simulink model "fine_delay_core"  (R2012b)
settings: Solver=ode45  StartTime=0.0  StopTime=10.0  RelTol=1e-3
libraries: xbsIndex_r4 x410, casper_library_misc x16, casper_library_multipliers x8
(part 2 of 4)

== system fine_delay_core/fd_fs0/fd_fs0/rotate0 ==
  sync : Inport
  x : Inport  Port=2
  a0 : Inport  Port=3
  a1 : Inport  Port=4
  din : Inport  Port=5
  Convert : xbsIndex_r4/Convert  gui_display_data_type=Fixed-point  arith_type="Signed  (2's comp)"  n_bits=data_bit_width  bin_pt=data_bit_width-1  float_type=Single  exp_bits=8  fraction_bits=24  quantization="Round  (unbiased: Even Values)"  overflow=Wrap  en=off  latency=conv_latency  dbl_ovrd=off  pipeline=on  block_type=convert
      settings: block_version=10.1.3
  Convert1 : xbsIndex_r4/Convert  gui_display_data_type=Fixed-point  arith_type="Signed  (2's comp)"  n_bits=data_bit_width  bin_pt=data_bit_width-1  float_type=Single  exp_bits=8  fraction_bits=24  quantization="Round  (unbiased: Even Values)"  overflow=Wrap  en=off  latency=conv_latency  dbl_ovrd=off  pipeline=on  block_type=convert
      settings: block_version=10.1.3
  Convert8 : xbsIndex_r4/Convert  gui_display_data_type=Fixed-point  arith_type="Signed  (2's comp)"  n_bits=lookup_bit_width  bin_pt=lookup_bit_width-1  float_type=Single  exp_bits=8  fraction_bits=24  quantization="Round  (unbiased: +/- Inf)"  overflow=Wrap  en=off  latency=conv_latency  dbl_ovrd=off  pipeline=on  block_type=convert
      settings: block_version=10.1.3
  Delay10 : xbsIndex_r4/Delay  rst=off  infoeditControl=Selection of Reset will increase slice count due to use of real FFs and instead of SRLs  en=off  latency=bram_latency  dbl_ovrd=off  reg_retiming=on  block_type=delay
  Delay13 : xbsIndex_r4/Delay  rst=off  infoeditControl=Selection of Reset will increase slice count due to use of real FFs and instead of SRLs  en=off  latency=conv_latency  dbl_ovrd=off  reg_retiming=on  block_type=delay
  Delay3 : xbsIndex_r4/Delay  rst=off  infoeditControl=Selection of Reset will increase slice count due to use of real FFs and instead of SRLs  en=off  latency=bram_latency  dbl_ovrd=off  reg_retiming=on  block_type=delay
  Delay6 : xbsIndex_r4/Delay  rst=off  infoeditControl=Selection of Reset will increase slice count due to use of real FFs and instead of SRLs  en=off  latency=mult_latency+add_latency+conv_latency  dbl_ovrd=off  reg_retiming=on  block_type=delay
  Delay9 : xbsIndex_r4/Delay  rst=off  infoeditControl=Selection of Reset will increase slice count due to use of real FFs and instead of SRLs  en=off  latency=add_latency+mult_latency+conv_latency  dbl_ovrd=off  reg_retiming=on  block_type=delay
  Reinterpret11 : xbsIndex_r4/Reinterpret  force_arith_type=on  arith_type=Unsigned  force_bin_pt=on  bin_pt=0  block_type=reinterpret
      settings: infoedit="Changes signal type without altering the binary representation.   You can changed the signal between signed and unsigned, and relocate the binary point.<br><br>Hardware notes: In hardware this block costs nothing.<br><br>Example:  Suppose the input is 6 bits wide, signed, with 2 fractional bits, and the output is forced to unsigned with 0 fractional bits.  Then an input of -2.0 (1110.00 in binary 2's complement) becomes an output of 56 (111000 in binary)."  block_version=10.1.3
  c_to_ri : casper_library_misc/c_to_ri  n_bits=data_bit_width  bin_pt=data_bit_width-1
  cmult_dsp48e : casper_library_multipliers/cmult_dsp48e  n_bits_a=18  bin_pt_a=17  n_bits_b=18  bin_pt_b=17  conjugated=off  full_precision=on  n_bits_c=37  bin_pt_c=34  quantization=Truncate  overflow=Wrap  cast_latency=0
      settings: AttributesFormatString=|
      | 18_17 * 18_17 ==> 37_34
      | Latency=4
  polynomial0 : Subsystem  mask(polynomial){order=1, mult_latency=mult_latency, add_latency=add_latency, bit_width_out=lookup_bit_width+fft_len, bin_pt_out=fft_len}
      mask prompts: order "Order of polynomial"; mult_latency "Multiplier latency"; add_latency "Add latency"; bit_width_out "Output bit width"; bin_pt_out "Output binary point"
      settings: AttributesFormatString=latency 6
  ri_to_c : casper_library_misc/ri_to_c
  sincos0 : Subsystem  AncestorBlock=casper_library_downconverter/sincos  mask(sincos){func=sine and cosine, neg_sin=off, neg_cos=off, symmetric=off, handle_sync=on, depth_bits=lookup_bit_width, bit_width=mix_bits, bram_latency=bram_latency}
      mask prompts: func "Function"; neg_sin "Negative sine"; neg_cos "Negative cosine"; symmetric "Symmetric output"; handle_sync "Handle sync"; depth_bits "Lookup table depth (2^?)"; bit_width "Output bit width"; bram_latency "BRAM latency"
      mask init:
      | sincos_init(gcb, ...
      |     'func', func, ...
      |     'neg_sin', neg_sin, ...
      |     'neg_cos', neg_cos, ...
      |     'symmetric', symmetric, ...
      |     'handle_sync', handle_sync, ...
      |     'depth_bits', depth_bits, ...
      |     'bit_width', bit_width, ...
      |     'bram_latency', bram_latency);
      mask TypeOptions func: cosine | sine | sine and cosine
  sync_out : Outport
  dout : Outport  Port=2
  wires:
  polynomial0/2(a0x^0+a1x^1) -> Convert8/1
  polynomial0/1(sync_out) -> Delay13/1
  Reinterpret11/1 -> sincos0/2(theta)
  sincos0/1(sync_out) -> Delay6/1
  cmult_dsp48e/1 -> Convert/1
  cmult_dsp48e/2 -> Convert1/1
  Convert/1 -> ri_to_c/1
  Convert1/1 -> ri_to_c/2
  sincos0/3(cos) -> cmult_dsp48e/1
  sincos0/2(sine) -> cmult_dsp48e/2
  c_to_ri/1 -> Delay10/1
  Delay10/1 -> cmult_dsp48e/3
  c_to_ri/2 -> Delay3/1
  Delay3/1 -> cmult_dsp48e/4
  Delay9/1 -> c_to_ri/1
  Delay13/1 -> sincos0/1(sync_in)
  Convert8/1 -> Reinterpret11/1
  sync/1 -> polynomial0/1(sync_in)
  Delay6/1 -> sync_out/1
  x/1 -> polynomial0/2(x)
  a0/1 -> polynomial0/3(a0)
  a1/1 -> polynomial0/4(a1)
  ri_to_c/1 -> dout/1
  din/1 -> Delay9/1

== system fine_delay_core/fd_fs0/fd_fs0/rotate1 ==
  sync : Inport
  x : Inport  Port=2
  a0 : Inport  Port=3
  a1 : Inport  Port=4
  din : Inport  Port=5
  Convert : xbsIndex_r4/Convert  gui_display_data_type=Fixed-point  arith_type="Signed  (2's comp)"  n_bits=data_bit_width  bin_pt=data_bit_width-1  float_type=Single  exp_bits=8  fraction_bits=24  quantization="Round  (unbiased: Even Values)"  overflow=Wrap  en=off  latency=conv_latency  dbl_ovrd=off  pipeline=on  block_type=convert
      settings: block_version=10.1.3
  Convert1 : xbsIndex_r4/Convert  gui_display_data_type=Fixed-point  arith_type="Signed  (2's comp)"  n_bits=data_bit_width  bin_pt=data_bit_width-1  float_type=Single  exp_bits=8  fraction_bits=24  quantization="Round  (unbiased: Even Values)"  overflow=Wrap  en=off  latency=conv_latency  dbl_ovrd=off  pipeline=on  block_type=convert
      settings: block_version=10.1.3
  Convert8 : xbsIndex_r4/Convert  gui_display_data_type=Fixed-point  arith_type="Signed  (2's comp)"  n_bits=lookup_bit_width  bin_pt=lookup_bit_width-1  float_type=Single  exp_bits=8  fraction_bits=24  quantization="Round  (unbiased: +/- Inf)"  overflow=Wrap  en=off  latency=conv_latency  dbl_ovrd=off  pipeline=on  block_type=convert
      settings: block_version=10.1.3
  Delay10 : xbsIndex_r4/Delay  rst=off  infoeditControl=Selection of Reset will increase slice count due to use of real FFs and instead of SRLs  en=off  latency=bram_latency  dbl_ovrd=off  reg_retiming=on  block_type=delay
  Delay13 : xbsIndex_r4/Delay  rst=off  infoeditControl=Selection of Reset will increase slice count due to use of real FFs and instead of SRLs  en=off  latency=conv_latency  dbl_ovrd=off  reg_retiming=on  block_type=delay
  Delay3 : xbsIndex_r4/Delay  rst=off  infoeditControl=Selection of Reset will increase slice count due to use of real FFs and instead of SRLs  en=off  latency=bram_latency  dbl_ovrd=off  reg_retiming=on  block_type=delay
  Delay6 : xbsIndex_r4/Delay  rst=off  infoeditControl=Selection of Reset will increase slice count due to use of real FFs and instead of SRLs  en=off  latency=mult_latency+add_latency+conv_latency  dbl_ovrd=off  reg_retiming=on  block_type=delay
  Delay9 : xbsIndex_r4/Delay  rst=off  infoeditControl=Selection of Reset will increase slice count due to use of real FFs and instead of SRLs  en=off  latency=add_latency+mult_latency+conv_latency  dbl_ovrd=off  reg_retiming=on  block_type=delay
  Reinterpret11 : xbsIndex_r4/Reinterpret  force_arith_type=on  arith_type=Unsigned  force_bin_pt=on  bin_pt=0  block_type=reinterpret
      settings: infoedit="Changes signal type without altering the binary representation.   You can changed the signal between signed and unsigned, and relocate the binary point.<br><br>Hardware notes: In hardware this block costs nothing.<br><br>Example:  Suppose the input is 6 bits wide, signed, with 2 fractional bits, and the output is forced to unsigned with 0 fractional bits.  Then an input of -2.0 (1110.00 in binary 2's complement) becomes an output of 56 (111000 in binary)."  block_version=10.1.3
  c_to_ri : casper_library_misc/c_to_ri  n_bits=data_bit_width  bin_pt=data_bit_width-1
  cmult_dsp48e : casper_library_multipliers/cmult_dsp48e  n_bits_a=18  bin_pt_a=17  n_bits_b=18  bin_pt_b=17  conjugated=off  full_precision=on  n_bits_c=37  bin_pt_c=34  quantization=Truncate  overflow=Wrap  cast_latency=0
      settings: AttributesFormatString=|
      | 18_17 * 18_17 ==> 37_34
      | Latency=4
  polynomial0 : Subsystem  mask(polynomial){order=1, mult_latency=mult_latency, add_latency=add_latency, bit_width_out=lookup_bit_width+fft_len, bin_pt_out=fft_len}
      mask prompts: order "Order of polynomial"; mult_latency "Multiplier latency"; add_latency "Add latency"; bit_width_out "Output bit width"; bin_pt_out "Output binary point"
      settings: AttributesFormatString=latency 6
  ri_to_c : casper_library_misc/ri_to_c
  sincos0 : Subsystem  AncestorBlock=casper_library_downconverter/sincos  mask(sincos){func=sine and cosine, neg_sin=off, neg_cos=off, symmetric=off, handle_sync=on, depth_bits=lookup_bit_width, bit_width=mix_bits, bram_latency=bram_latency}
      mask prompts: func "Function"; neg_sin "Negative sine"; neg_cos "Negative cosine"; symmetric "Symmetric output"; handle_sync "Handle sync"; depth_bits "Lookup table depth (2^?)"; bit_width "Output bit width"; bram_latency "BRAM latency"
      mask init: same as fine_delay_core/fd_fs0/fd_fs0/rotate0/sincos0
      mask TypeOptions func: cosine | sine | sine and cosine
  sync_out : Outport
  dout : Outport  Port=2
  wires:
  din/1 -> Delay9/1
  ri_to_c/1 -> dout/1
  a1/1 -> polynomial0/4(a1)
  a0/1 -> polynomial0/3(a0)
  x/1 -> polynomial0/2(x)
  Delay6/1 -> sync_out/1
  sync/1 -> polynomial0/1(sync_in)
  Convert8/1 -> Reinterpret11/1
  Delay13/1 -> sincos0/1(sync_in)
  Delay9/1 -> c_to_ri/1
  Delay3/1 -> cmult_dsp48e/4
  c_to_ri/2 -> Delay3/1
  Delay10/1 -> cmult_dsp48e/3
  c_to_ri/1 -> Delay10/1
  sincos0/2(sine) -> cmult_dsp48e/2
  sincos0/3(cos) -> cmult_dsp48e/1
  Convert1/1 -> ri_to_c/2
  Convert/1 -> ri_to_c/1
  cmult_dsp48e/2 -> Convert1/1
  cmult_dsp48e/1 -> Convert/1
  sincos0/1(sync_out) -> Delay6/1
  Reinterpret11/1 -> sincos0/2(theta)
  polynomial0/1(sync_out) -> Delay13/1
  polynomial0/2(a0x^0+a1x^1) -> Convert8/1

== system fine_delay_core/fd_fs0/fd_fs0/rotate2 ==
  sync : Inport
  x : Inport  Port=2
  a0 : Inport  Port=3
  a1 : Inport  Port=4
  din : Inport  Port=5
  Convert : xbsIndex_r4/Convert  gui_display_data_type=Fixed-point  arith_type="Signed  (2's comp)"  n_bits=data_bit_width  bin_pt=data_bit_width-1  float_type=Single  exp_bits=8  fraction_bits=24  quantization="Round  (unbiased: Even Values)"  overflow=Wrap  en=off  latency=conv_latency  dbl_ovrd=off  pipeline=on  block_type=convert
      settings: block_version=10.1.3
  Convert1 : xbsIndex_r4/Convert  gui_display_data_type=Fixed-point  arith_type="Signed  (2's comp)"  n_bits=data_bit_width  bin_pt=data_bit_width-1  float_type=Single  exp_bits=8  fraction_bits=24  quantization="Round  (unbiased: Even Values)"  overflow=Wrap  en=off  latency=conv_latency  dbl_ovrd=off  pipeline=on  block_type=convert
      settings: block_version=10.1.3
  Convert8 : xbsIndex_r4/Convert  gui_display_data_type=Fixed-point  arith_type="Signed  (2's comp)"  n_bits=lookup_bit_width  bin_pt=lookup_bit_width-1  float_type=Single  exp_bits=8  fraction_bits=24  quantization="Round  (unbiased: +/- Inf)"  overflow=Wrap  en=off  latency=conv_latency  dbl_ovrd=off  pipeline=on  block_type=convert
      settings: block_version=10.1.3
  Delay10 : xbsIndex_r4/Delay  rst=off  infoeditControl=Selection of Reset will increase slice count due to use of real FFs and instead of SRLs  en=off  latency=bram_latency  dbl_ovrd=off  reg_retiming=on  block_type=delay
  Delay13 : xbsIndex_r4/Delay  rst=off  infoeditControl=Selection of Reset will increase slice count due to use of real FFs and instead of SRLs  en=off  latency=conv_latency  dbl_ovrd=off  reg_retiming=on  block_type=delay
  Delay3 : xbsIndex_r4/Delay  rst=off  infoeditControl=Selection of Reset will increase slice count due to use of real FFs and instead of SRLs  en=off  latency=bram_latency  dbl_ovrd=off  reg_retiming=on  block_type=delay
  Delay6 : xbsIndex_r4/Delay  rst=off  infoeditControl=Selection of Reset will increase slice count due to use of real FFs and instead of SRLs  en=off  latency=mult_latency+add_latency+conv_latency  dbl_ovrd=off  reg_retiming=on  block_type=delay
  Delay9 : xbsIndex_r4/Delay  rst=off  infoeditControl=Selection of Reset will increase slice count due to use of real FFs and instead of SRLs  en=off  latency=add_latency+mult_latency+conv_latency  dbl_ovrd=off  reg_retiming=on  block_type=delay
  Reinterpret11 : xbsIndex_r4/Reinterpret  force_arith_type=on  arith_type=Unsigned  force_bin_pt=on  bin_pt=0  block_type=reinterpret
      settings: infoedit="Changes signal type without altering the binary representation.   You can changed the signal between signed and unsigned, and relocate the binary point.<br><br>Hardware notes: In hardware this block costs nothing.<br><br>Example:  Suppose the input is 6 bits wide, signed, with 2 fractional bits, and the output is forced to unsigned with 0 fractional bits.  Then an input of -2.0 (1110.00 in binary 2's complement) becomes an output of 56 (111000 in binary)."  block_version=10.1.3
  c_to_ri : casper_library_misc/c_to_ri  n_bits=data_bit_width  bin_pt=data_bit_width-1
  cmult_dsp48e : casper_library_multipliers/cmult_dsp48e  n_bits_a=18  bin_pt_a=17  n_bits_b=18  bin_pt_b=17  conjugated=off  full_precision=on  n_bits_c=37  bin_pt_c=34  quantization=Truncate  overflow=Wrap  cast_latency=0
      settings: AttributesFormatString=|
      | 18_17 * 18_17 ==> 37_34
      | Latency=4
  polynomial0 : Subsystem  mask(polynomial){order=1, mult_latency=mult_latency, add_latency=add_latency, bit_width_out=lookup_bit_width+fft_len, bin_pt_out=fft_len}
      mask prompts: order "Order of polynomial"; mult_latency "Multiplier latency"; add_latency "Add latency"; bit_width_out "Output bit width"; bin_pt_out "Output binary point"
      settings: AttributesFormatString=latency 6
  ri_to_c : casper_library_misc/ri_to_c
  sincos0 : Subsystem  AncestorBlock=casper_library_downconverter/sincos  mask(sincos){func=sine and cosine, neg_sin=off, neg_cos=off, symmetric=off, handle_sync=on, depth_bits=lookup_bit_width, bit_width=mix_bits, bram_latency=bram_latency}
      mask prompts: func "Function"; neg_sin "Negative sine"; neg_cos "Negative cosine"; symmetric "Symmetric output"; handle_sync "Handle sync"; depth_bits "Lookup table depth (2^?)"; bit_width "Output bit width"; bram_latency "BRAM latency"
      mask init: same as fine_delay_core/fd_fs0/fd_fs0/rotate0/sincos0
      mask TypeOptions func: cosine | sine | sine and cosine
  sync_out : Outport
  dout : Outport  Port=2
  wires:
  din/1 -> Delay9/1
  ri_to_c/1 -> dout/1
  a1/1 -> polynomial0/4(a1)
  a0/1 -> polynomial0/3(a0)
  x/1 -> polynomial0/2(x)
  Delay6/1 -> sync_out/1
  sync/1 -> polynomial0/1(sync_in)
  Convert8/1 -> Reinterpret11/1
  Delay13/1 -> sincos0/1(sync_in)
  Delay9/1 -> c_to_ri/1
  Delay3/1 -> cmult_dsp48e/4
  c_to_ri/2 -> Delay3/1
  Delay10/1 -> cmult_dsp48e/3
  c_to_ri/1 -> Delay10/1
  sincos0/2(sine) -> cmult_dsp48e/2
  sincos0/3(cos) -> cmult_dsp48e/1
  Convert1/1 -> ri_to_c/2
  Convert/1 -> ri_to_c/1
  cmult_dsp48e/2 -> Convert1/1
  cmult_dsp48e/1 -> Convert/1
  sincos0/1(sync_out) -> Delay6/1
  Reinterpret11/1 -> sincos0/2(theta)
  polynomial0/1(sync_out) -> Delay13/1
  polynomial0/2(a0x^0+a1x^1) -> Convert8/1

== system fine_delay_core/fd_fs0/fd_fs0/rotate3 ==
  sync : Inport
  x : Inport  Port=2
  a0 : Inport  Port=3
  a1 : Inport  Port=4
  din : Inport  Port=5
  Convert : xbsIndex_r4/Convert  gui_display_data_type=Fixed-point  arith_type="Signed  (2's comp)"  n_bits=data_bit_width  bin_pt=data_bit_width-1  float_type=Single  exp_bits=8  fraction_bits=24  quantization="Round  (unbiased: Even Values)"  overflow=Wrap  en=off  latency=conv_latency  dbl_ovrd=off  pipeline=on  block_type=convert
      settings: block_version=10.1.3
  Convert1 : xbsIndex_r4/Convert  gui_display_data_type=Fixed-point  arith_type="Signed  (2's comp)"  n_bits=data_bit_width  bin_pt=data_bit_width-1  float_type=Single  exp_bits=8  fraction_bits=24  quantization="Round  (unbiased: Even Values)"  overflow=Wrap  en=off  latency=conv_latency  dbl_ovrd=off  pipeline=on  block_type=convert
      settings: block_version=10.1.3
  Convert8 : xbsIndex_r4/Convert  gui_display_data_type=Fixed-point  arith_type="Signed  (2's comp)"  n_bits=lookup_bit_width  bin_pt=lookup_bit_width-1  float_type=Single  exp_bits=8  fraction_bits=24  quantization="Round  (unbiased: +/- Inf)"  overflow=Wrap  en=off  latency=conv_latency  dbl_ovrd=off  pipeline=on  block_type=convert
      settings: block_version=10.1.3
  Delay10 : xbsIndex_r4/Delay  rst=off  infoeditControl=Selection of Reset will increase slice count due to use of real FFs and instead of SRLs  en=off  latency=bram_latency  dbl_ovrd=off  reg_retiming=on  block_type=delay
  Delay13 : xbsIndex_r4/Delay  rst=off  infoeditControl=Selection of Reset will increase slice count due to use of real FFs and instead of SRLs  en=off  latency=conv_latency  dbl_ovrd=off  reg_retiming=on  block_type=delay
  Delay3 : xbsIndex_r4/Delay  rst=off  infoeditControl=Selection of Reset will increase slice count due to use of real FFs and instead of SRLs  en=off  latency=bram_latency  dbl_ovrd=off  reg_retiming=on  block_type=delay
  Delay6 : xbsIndex_r4/Delay  rst=off  infoeditControl=Selection of Reset will increase slice count due to use of real FFs and instead of SRLs  en=off  latency=mult_latency+add_latency+conv_latency  dbl_ovrd=off  reg_retiming=on  block_type=delay
  Delay9 : xbsIndex_r4/Delay  rst=off  infoeditControl=Selection of Reset will increase slice count due to use of real FFs and instead of SRLs  en=off  latency=add_latency+mult_latency+conv_latency  dbl_ovrd=off  reg_retiming=on  block_type=delay
  Reinterpret11 : xbsIndex_r4/Reinterpret  force_arith_type=on  arith_type=Unsigned  force_bin_pt=on  bin_pt=0  block_type=reinterpret
      settings: infoedit="Changes signal type without altering the binary representation.   You can changed the signal between signed and unsigned, and relocate the binary point.<br><br>Hardware notes: In hardware this block costs nothing.<br><br>Example:  Suppose the input is 6 bits wide, signed, with 2 fractional bits, and the output is forced to unsigned with 0 fractional bits.  Then an input of -2.0 (1110.00 in binary 2's complement) becomes an output of 56 (111000 in binary)."  block_version=10.1.3
  c_to_ri : casper_library_misc/c_to_ri  n_bits=data_bit_width  bin_pt=data_bit_width-1
  cmult_dsp48e : casper_library_multipliers/cmult_dsp48e  n_bits_a=18  bin_pt_a=17  n_bits_b=18  bin_pt_b=17  conjugated=off  full_precision=on  n_bits_c=37  bin_pt_c=34  quantization=Truncate  overflow=Wrap  cast_latency=0
      settings: AttributesFormatString=|
      | 18_17 * 18_17 ==> 37_34
      | Latency=4
  polynomial0 : Subsystem  mask(polynomial){order=1, mult_latency=mult_latency, add_latency=add_latency, bit_width_out=lookup_bit_width+fft_len, bin_pt_out=fft_len}
      mask prompts: order "Order of polynomial"; mult_latency "Multiplier latency"; add_latency "Add latency"; bit_width_out "Output bit width"; bin_pt_out "Output binary point"
      settings: AttributesFormatString=latency 6
  ri_to_c : casper_library_misc/ri_to_c
  sincos0 : Subsystem  AncestorBlock=casper_library_downconverter/sincos  mask(sincos){func=sine and cosine, neg_sin=off, neg_cos=off, symmetric=off, handle_sync=on, depth_bits=lookup_bit_width, bit_width=mix_bits, bram_latency=bram_latency}
      mask prompts: func "Function"; neg_sin "Negative sine"; neg_cos "Negative cosine"; symmetric "Symmetric output"; handle_sync "Handle sync"; depth_bits "Lookup table depth (2^?)"; bit_width "Output bit width"; bram_latency "BRAM latency"
      mask init: same as fine_delay_core/fd_fs0/fd_fs0/rotate0/sincos0
      mask TypeOptions func: cosine | sine | sine and cosine
  sync_out : Outport
  dout : Outport  Port=2
  wires:
  polynomial0/2(a0x^0+a1x^1) -> Convert8/1
  polynomial0/1(sync_out) -> Delay13/1
  Reinterpret11/1 -> sincos0/2(theta)
  sincos0/1(sync_out) -> Delay6/1
  cmult_dsp48e/1 -> Convert/1
  cmult_dsp48e/2 -> Convert1/1
  Convert/1 -> ri_to_c/1
  Convert1/1 -> ri_to_c/2
  sincos0/3(cos) -> cmult_dsp48e/1
  sincos0/2(sine) -> cmult_dsp48e/2
  c_to_ri/1 -> Delay10/1
  Delay10/1 -> cmult_dsp48e/3
  c_to_ri/2 -> Delay3/1
  Delay3/1 -> cmult_dsp48e/4
  Delay9/1 -> c_to_ri/1
  Delay13/1 -> sincos0/1(sync_in)
  Convert8/1 -> Reinterpret11/1
  sync/1 -> polynomial0/1(sync_in)
  Delay6/1 -> sync_out/1
  x/1 -> polynomial0/2(x)
  a0/1 -> polynomial0/3(a0)
  a1/1 -> polynomial0/4(a1)
  ri_to_c/1 -> dout/1
  din/1 -> Delay9/1

== system fine_delay_core/fd_fs0/fd_fs0/rotate4 ==
  sync : Inport
  x : Inport  Port=2
  a0 : Inport  Port=3
  a1 : Inport  Port=4
  din : Inport  Port=5
  Convert : xbsIndex_r4/Convert  gui_display_data_type=Fixed-point  arith_type="Signed  (2's comp)"  n_bits=data_bit_width  bin_pt=data_bit_width-1  float_type=Single  exp_bits=8  fraction_bits=24  quantization="Round  (unbiased: Even Values)"  overflow=Wrap  en=off  latency=conv_latency  dbl_ovrd=off  pipeline=on  block_type=convert
      settings: block_version=10.1.3
  Convert1 : xbsIndex_r4/Convert  gui_display_data_type=Fixed-point  arith_type="Signed  (2's comp)"  n_bits=data_bit_width  bin_pt=data_bit_width-1  float_type=Single  exp_bits=8  fraction_bits=24  quantization="Round  (unbiased: Even Values)"  overflow=Wrap  en=off  latency=conv_latency  dbl_ovrd=off  pipeline=on  block_type=convert
      settings: block_version=10.1.3
  Convert8 : xbsIndex_r4/Convert  gui_display_data_type=Fixed-point  arith_type="Signed  (2's comp)"  n_bits=lookup_bit_width  bin_pt=lookup_bit_width-1  float_type=Single  exp_bits=8  fraction_bits=24  quantization="Round  (unbiased: +/- Inf)"  overflow=Wrap  en=off  latency=conv_latency  dbl_ovrd=off  pipeline=on  block_type=convert
      settings: block_version=10.1.3
  Delay10 : xbsIndex_r4/Delay  rst=off  infoeditControl=Selection of Reset will increase slice count due to use of real FFs and instead of SRLs  en=off  latency=bram_latency  dbl_ovrd=off  reg_retiming=on  block_type=delay
  Delay13 : xbsIndex_r4/Delay  rst=off  infoeditControl=Selection of Reset will increase slice count due to use of real FFs and instead of SRLs  en=off  latency=conv_latency  dbl_ovrd=off  reg_retiming=on  block_type=delay
  Delay3 : xbsIndex_r4/Delay  rst=off  infoeditControl=Selection of Reset will increase slice count due to use of real FFs and instead of SRLs  en=off  latency=bram_latency  dbl_ovrd=off  reg_retiming=on  block_type=delay
  Delay6 : xbsIndex_r4/Delay  rst=off  infoeditControl=Selection of Reset will increase slice count due to use of real FFs and instead of SRLs  en=off  latency=mult_latency+add_latency+conv_latency  dbl_ovrd=off  reg_retiming=on  block_type=delay
  Delay9 : xbsIndex_r4/Delay  rst=off  infoeditControl=Selection of Reset will increase slice count due to use of real FFs and instead of SRLs  en=off  latency=add_latency+mult_latency+conv_latency  dbl_ovrd=off  reg_retiming=on  block_type=delay
  Reinterpret11 : xbsIndex_r4/Reinterpret  force_arith_type=on  arith_type=Unsigned  force_bin_pt=on  bin_pt=0  block_type=reinterpret
      settings: infoedit="Changes signal type without altering the binary representation.   You can changed the signal between signed and unsigned, and relocate the binary point.<br><br>Hardware notes: In hardware this block costs nothing.<br><br>Example:  Suppose the input is 6 bits wide, signed, with 2 fractional bits, and the output is forced to unsigned with 0 fractional bits.  Then an input of -2.0 (1110.00 in binary 2's complement) becomes an output of 56 (111000 in binary)."  block_version=10.1.3
  c_to_ri : casper_library_misc/c_to_ri  n_bits=data_bit_width  bin_pt=data_bit_width-1
  cmult_dsp48e : casper_library_multipliers/cmult_dsp48e  n_bits_a=18  bin_pt_a=17  n_bits_b=18  bin_pt_b=17  conjugated=off  full_precision=on  n_bits_c=37  bin_pt_c=34  quantization=Truncate  overflow=Wrap  cast_latency=0
      settings: AttributesFormatString=|
      | 18_17 * 18_17 ==> 37_34
      | Latency=4
  polynomial0 : Subsystem  mask(polynomial){order=1, mult_latency=mult_latency, add_latency=add_latency, bit_width_out=lookup_bit_width+fft_len, bin_pt_out=fft_len}
      mask prompts: order "Order of polynomial"; mult_latency "Multiplier latency"; add_latency "Add latency"; bit_width_out "Output bit width"; bin_pt_out "Output binary point"
      settings: AttributesFormatString=latency 6
  ri_to_c : casper_library_misc/ri_to_c
  sincos0 : Subsystem  AncestorBlock=casper_library_downconverter/sincos  mask(sincos){func=sine and cosine, neg_sin=off, neg_cos=off, symmetric=off, handle_sync=on, depth_bits=lookup_bit_width, bit_width=mix_bits, bram_latency=bram_latency}
      mask prompts: func "Function"; neg_sin "Negative sine"; neg_cos "Negative cosine"; symmetric "Symmetric output"; handle_sync "Handle sync"; depth_bits "Lookup table depth (2^?)"; bit_width "Output bit width"; bram_latency "BRAM latency"
      mask init: same as fine_delay_core/fd_fs0/fd_fs0/rotate0/sincos0
      mask TypeOptions func: cosine | sine | sine and cosine
  sync_out : Outport
  dout : Outport  Port=2
  wires:
  polynomial0/2(a0x^0+a1x^1) -> Convert8/1
  polynomial0/1(sync_out) -> Delay13/1
  Reinterpret11/1 -> sincos0/2(theta)
  sincos0/1(sync_out) -> Delay6/1
  cmult_dsp48e/1 -> Convert/1
  cmult_dsp48e/2 -> Convert1/1
  Convert/1 -> ri_to_c/1
  Convert1/1 -> ri_to_c/2
  sincos0/3(cos) -> cmult_dsp48e/1
  sincos0/2(sine) -> cmult_dsp48e/2
  c_to_ri/1 -> Delay10/1
  Delay10/1 -> cmult_dsp48e/3
  c_to_ri/2 -> Delay3/1
  Delay3/1 -> cmult_dsp48e/4
  Delay9/1 -> c_to_ri/1
  Delay13/1 -> sincos0/1(sync_in)
  Convert8/1 -> Reinterpret11/1
  sync/1 -> polynomial0/1(sync_in)
  Delay6/1 -> sync_out/1
  x/1 -> polynomial0/2(x)
  a0/1 -> polynomial0/3(a0)
  a1/1 -> polynomial0/4(a1)
  ri_to_c/1 -> dout/1
  din/1 -> Delay9/1

== system fine_delay_core/fd_fs0/fd_fs0/rotate5 ==
  sync : Inport
  x : Inport  Port=2
  a0 : Inport  Port=3
  a1 : Inport  Port=4
  din : Inport  Port=5
  Convert : xbsIndex_r4/Convert  gui_display_data_type=Fixed-point  arith_type="Signed  (2's comp)"  n_bits=data_bit_width  bin_pt=data_bit_width-1  float_type=Single  exp_bits=8  fraction_bits=24  quantization="Round  (unbiased: Even Values)"  overflow=Wrap  en=off  latency=conv_latency  dbl_ovrd=off  pipeline=on  block_type=convert
      settings: block_version=10.1.3
  Convert1 : xbsIndex_r4/Convert  gui_display_data_type=Fixed-point  arith_type="Signed  (2's comp)"  n_bits=data_bit_width  bin_pt=data_bit_width-1  float_type=Single  exp_bits=8  fraction_bits=24  quantization="Round  (unbiased: Even Values)"  overflow=Wrap  en=off  latency=conv_latency  dbl_ovrd=off  pipeline=on  block_type=convert
      settings: block_version=10.1.3
  Convert8 : xbsIndex_r4/Convert  gui_display_data_type=Fixed-point  arith_type="Signed  (2's comp)"  n_bits=lookup_bit_width  bin_pt=lookup_bit_width-1  float_type=Single  exp_bits=8  fraction_bits=24  quantization="Round  (unbiased: +/- Inf)"  overflow=Wrap  en=off  latency=conv_latency  dbl_ovrd=off  pipeline=on  block_type=convert
      settings: block_version=10.1.3
  Delay10 : xbsIndex_r4/Delay  rst=off  infoeditControl=Selection of Reset will increase slice count due to use of real FFs and instead of SRLs  en=off  latency=bram_latency  dbl_ovrd=off  reg_retiming=on  block_type=delay
  Delay13 : xbsIndex_r4/Delay  rst=off  infoeditControl=Selection of Reset will increase slice count due to use of real FFs and instead of SRLs  en=off  latency=conv_latency  dbl_ovrd=off  reg_retiming=on  block_type=delay
  Delay3 : xbsIndex_r4/Delay  rst=off  infoeditControl=Selection of Reset will increase slice count due to use of real FFs and instead of SRLs  en=off  latency=bram_latency  dbl_ovrd=off  reg_retiming=on  block_type=delay
  Delay6 : xbsIndex_r4/Delay  rst=off  infoeditControl=Selection of Reset will increase slice count due to use of real FFs and instead of SRLs  en=off  latency=mult_latency+add_latency+conv_latency  dbl_ovrd=off  reg_retiming=on  block_type=delay
  Delay9 : xbsIndex_r4/Delay  rst=off  infoeditControl=Selection of Reset will increase slice count due to use of real FFs and instead of SRLs  en=off  latency=add_latency+mult_latency+conv_latency  dbl_ovrd=off  reg_retiming=on  block_type=delay
  Reinterpret11 : xbsIndex_r4/Reinterpret  force_arith_type=on  arith_type=Unsigned  force_bin_pt=on  bin_pt=0  block_type=reinterpret
      settings: infoedit="Changes signal type without altering the binary representation.   You can changed the signal between signed and unsigned, and relocate the binary point.<br><br>Hardware notes: In hardware this block costs nothing.<br><br>Example:  Suppose the input is 6 bits wide, signed, with 2 fractional bits, and the output is forced to unsigned with 0 fractional bits.  Then an input of -2.0 (1110.00 in binary 2's complement) becomes an output of 56 (111000 in binary)."  block_version=10.1.3
  c_to_ri : casper_library_misc/c_to_ri  n_bits=data_bit_width  bin_pt=data_bit_width-1
  cmult_dsp48e : casper_library_multipliers/cmult_dsp48e  n_bits_a=18  bin_pt_a=17  n_bits_b=18  bin_pt_b=17  conjugated=off  full_precision=on  n_bits_c=37  bin_pt_c=34  quantization=Truncate  overflow=Wrap  cast_latency=0
      settings: AttributesFormatString=|
      | 18_17 * 18_17 ==> 37_34
      | Latency=4
  polynomial0 : Subsystem  mask(polynomial){order=1, mult_latency=mult_latency, add_latency=add_latency, bit_width_out=lookup_bit_width+fft_len, bin_pt_out=fft_len}
      mask prompts: order "Order of polynomial"; mult_latency "Multiplier latency"; add_latency "Add latency"; bit_width_out "Output bit width"; bin_pt_out "Output binary point"
      settings: AttributesFormatString=latency 6
  ri_to_c : casper_library_misc/ri_to_c
  sincos0 : Subsystem  AncestorBlock=casper_library_downconverter/sincos  mask(sincos){func=sine and cosine, neg_sin=off, neg_cos=off, symmetric=off, handle_sync=on, depth_bits=lookup_bit_width, bit_width=mix_bits, bram_latency=bram_latency}
      mask prompts: func "Function"; neg_sin "Negative sine"; neg_cos "Negative cosine"; symmetric "Symmetric output"; handle_sync "Handle sync"; depth_bits "Lookup table depth (2^?)"; bit_width "Output bit width"; bram_latency "BRAM latency"
      mask init: same as fine_delay_core/fd_fs0/fd_fs0/rotate0/sincos0
      mask TypeOptions func: cosine | sine | sine and cosine
  sync_out : Outport
  dout : Outport  Port=2
  wires:
  din/1 -> Delay9/1
  ri_to_c/1 -> dout/1
  a1/1 -> polynomial0/4(a1)
  a0/1 -> polynomial0/3(a0)
  x/1 -> polynomial0/2(x)
  Delay6/1 -> sync_out/1
  sync/1 -> polynomial0/1(sync_in)
  Convert8/1 -> Reinterpret11/1
  Delay13/1 -> sincos0/1(sync_in)
  Delay9/1 -> c_to_ri/1
  Delay3/1 -> cmult_dsp48e/4
  c_to_ri/2 -> Delay3/1
  Delay10/1 -> cmult_dsp48e/3
  c_to_ri/1 -> Delay10/1
  sincos0/2(sine) -> cmult_dsp48e/2
  sincos0/3(cos) -> cmult_dsp48e/1
  Convert1/1 -> ri_to_c/2
  Convert/1 -> ri_to_c/1
  cmult_dsp48e/2 -> Convert1/1
  cmult_dsp48e/1 -> Convert/1
  sincos0/1(sync_out) -> Delay6/1
  Reinterpret11/1 -> sincos0/2(theta)
  polynomial0/1(sync_out) -> Delay13/1
  polynomial0/2(a0x^0+a1x^1) -> Convert8/1

== system fine_delay_core/fd_fs0/fd_fs0/rotate6 ==
  sync : Inport
  x : Inport  Port=2
  a0 : Inport  Port=3
  a1 : Inport  Port=4
  din : Inport  Port=5
  Convert : xbsIndex_r4/Convert  gui_display_data_type=Fixed-point  arith_type="Signed  (2's comp)"  n_bits=data_bit_width  bin_pt=data_bit_width-1  float_type=Single  exp_bits=8  fraction_bits=24  quantization="Round  (unbiased: Even Values)"  overflow=Wrap  en=off  latency=conv_latency  dbl_ovrd=off  pipeline=on  block_type=convert
      settings: block_version=10.1.3
  Convert1 : xbsIndex_r4/Convert  gui_display_data_type=Fixed-point  arith_type="Signed  (2's comp)"  n_bits=data_bit_width  bin_pt=data_bit_width-1  float_type=Single  exp_bits=8  fraction_bits=24  quantization="Round  (unbiased: Even Values)"  overflow=Wrap  en=off  latency=conv_latency  dbl_ovrd=off  pipeline=on  block_type=convert
      settings: block_version=10.1.3
  Convert8 : xbsIndex_r4/Convert  gui_display_data_type=Fixed-point  arith_type="Signed  (2's comp)"  n_bits=lookup_bit_width  bin_pt=lookup_bit_width-1  float_type=Single  exp_bits=8  fraction_bits=24  quantization="Round  (unbiased: +/- Inf)"  overflow=Wrap  en=off  latency=conv_latency  dbl_ovrd=off  pipeline=on  block_type=convert
      settings: block_version=10.1.3
  Delay10 : xbsIndex_r4/Delay  rst=off  infoeditControl=Selection of Reset will increase slice count due to use of real FFs and instead of SRLs  en=off  latency=bram_latency  dbl_ovrd=off  reg_retiming=on  block_type=delay
  Delay13 : xbsIndex_r4/Delay  rst=off  infoeditControl=Selection of Reset will increase slice count due to use of real FFs and instead of SRLs  en=off  latency=conv_latency  dbl_ovrd=off  reg_retiming=on  block_type=delay
  Delay3 : xbsIndex_r4/Delay  rst=off  infoeditControl=Selection of Reset will increase slice count due to use of real FFs and instead of SRLs  en=off  latency=bram_latency  dbl_ovrd=off  reg_retiming=on  block_type=delay
  Delay6 : xbsIndex_r4/Delay  rst=off  infoeditControl=Selection of Reset will increase slice count due to use of real FFs and instead of SRLs  en=off  latency=mult_latency+add_latency+conv_latency  dbl_ovrd=off  reg_retiming=on  block_type=delay
  Delay9 : xbsIndex_r4/Delay  rst=off  infoeditControl=Selection of Reset will increase slice count due to use of real FFs and instead of SRLs  en=off  latency=add_latency+mult_latency+conv_latency  dbl_ovrd=off  reg_retiming=on  block_type=delay
  Reinterpret11 : xbsIndex_r4/Reinterpret  force_arith_type=on  arith_type=Unsigned  force_bin_pt=on  bin_pt=0  block_type=reinterpret
      settings: infoedit="Changes signal type without altering the binary representation.   You can changed the signal between signed and unsigned, and relocate the binary point.<br><br>Hardware notes: In hardware this block costs nothing.<br><br>Example:  Suppose the input is 6 bits wide, signed, with 2 fractional bits, and the output is forced to unsigned with 0 fractional bits.  Then an input of -2.0 (1110.00 in binary 2's complement) becomes an output of 56 (111000 in binary)."  block_version=10.1.3
  c_to_ri : casper_library_misc/c_to_ri  n_bits=data_bit_width  bin_pt=data_bit_width-1
  cmult_dsp48e : casper_library_multipliers/cmult_dsp48e  n_bits_a=18  bin_pt_a=17  n_bits_b=18  bin_pt_b=17  conjugated=off  full_precision=on  n_bits_c=37  bin_pt_c=34  quantization=Truncate  overflow=Wrap  cast_latency=0
      settings: AttributesFormatString=|
      | 18_17 * 18_17 ==> 37_34
      | Latency=4
  polynomial0 : Subsystem  mask(polynomial){order=1, mult_latency=mult_latency, add_latency=add_latency, bit_width_out=lookup_bit_width+fft_len, bin_pt_out=fft_len}
      mask prompts: order "Order of polynomial"; mult_latency "Multiplier latency"; add_latency "Add latency"; bit_width_out "Output bit width"; bin_pt_out "Output binary point"
      settings: AttributesFormatString=latency 6
  ri_to_c : casper_library_misc/ri_to_c
  sincos0 : Subsystem  AncestorBlock=casper_library_downconverter/sincos  mask(sincos){func=sine and cosine, neg_sin=off, neg_cos=off, symmetric=off, handle_sync=on, depth_bits=lookup_bit_width, bit_width=mix_bits, bram_latency=bram_latency}
      mask prompts: func "Function"; neg_sin "Negative sine"; neg_cos "Negative cosine"; symmetric "Symmetric output"; handle_sync "Handle sync"; depth_bits "Lookup table depth (2^?)"; bit_width "Output bit width"; bram_latency "BRAM latency"
      mask init: same as fine_delay_core/fd_fs0/fd_fs0/rotate0/sincos0
      mask TypeOptions func: cosine | sine | sine and cosine
  sync_out : Outport
  dout : Outport  Port=2
  wires:
  din/1 -> Delay9/1
  ri_to_c/1 -> dout/1
  a1/1 -> polynomial0/4(a1)
  a0/1 -> polynomial0/3(a0)
  x/1 -> polynomial0/2(x)
  Delay6/1 -> sync_out/1
  sync/1 -> polynomial0/1(sync_in)
  Convert8/1 -> Reinterpret11/1
  Delay13/1 -> sincos0/1(sync_in)
  Delay9/1 -> c_to_ri/1
  Delay3/1 -> cmult_dsp48e/4
  c_to_ri/2 -> Delay3/1
  Delay10/1 -> cmult_dsp48e/3
  c_to_ri/1 -> Delay10/1
  sincos0/2(sine) -> cmult_dsp48e/2
  sincos0/3(cos) -> cmult_dsp48e/1
  Convert1/1 -> ri_to_c/2
  Convert/1 -> ri_to_c/1
  cmult_dsp48e/2 -> Convert1/1
  cmult_dsp48e/1 -> Convert/1
  sincos0/1(sync_out) -> Delay6/1
  Reinterpret11/1 -> sincos0/2(theta)
  polynomial0/1(sync_out) -> Delay13/1
  polynomial0/2(a0x^0+a1x^1) -> Convert8/1

== system fine_delay_core/fd_fs0/fd_fs0/rotate7 ==
  sync : Inport
  x : Inport  Port=2
  a0 : Inport  Port=3
  a1 : Inport  Port=4
  din : Inport  Port=5
  Convert : xbsIndex_r4/Convert  gui_display_data_type=Fixed-point  arith_type="Signed  (2's comp)"  n_bits=data_bit_width  bin_pt=data_bit_width-1  float_type=Single  exp_bits=8  fraction_bits=24  quantization="Round  (unbiased: Even Values)"  overflow=Wrap  en=off  latency=conv_latency  dbl_ovrd=off  pipeline=on  block_type=convert
      settings: block_version=10.1.3
  Convert1 : xbsIndex_r4/Convert  gui_display_data_type=Fixed-point  arith_type="Signed  (2's comp)"  n_bits=data_bit_width  bin_pt=data_bit_width-1  float_type=Single  exp_bits=8  fraction_bits=24  quantization="Round  (unbiased: Even Values)"  overflow=Wrap  en=off  latency=conv_latency  dbl_ovrd=off  pipeline=on  block_type=convert
      settings: block_version=10.1.3
  Convert8 : xbsIndex_r4/Convert  gui_display_data_type=Fixed-point  arith_type="Signed  (2's comp)"  n_bits=lookup_bit_width  bin_pt=lookup_bit_width-1  float_type=Single  exp_bits=8  fraction_bits=24  quantization="Round  (unbiased: +/- Inf)"  overflow=Wrap  en=off  latency=conv_latency  dbl_ovrd=off  pipeline=on  block_type=convert
      settings: block_version=10.1.3
  Delay10 : xbsIndex_r4/Delay  rst=off  infoeditControl=Selection of Reset will increase slice count due to use of real FFs and instead of SRLs  en=off  latency=bram_latency  dbl_ovrd=off  reg_retiming=on  block_type=delay
  Delay13 : xbsIndex_r4/Delay  rst=off  infoeditControl=Selection of Reset will increase slice count due to use of real FFs and instead of SRLs  en=off  latency=conv_latency  dbl_ovrd=off  reg_retiming=on  block_type=delay
  Delay3 : xbsIndex_r4/Delay  rst=off  infoeditControl=Selection of Reset will increase slice count due to use of real FFs and instead of SRLs  en=off  latency=bram_latency  dbl_ovrd=off  reg_retiming=on  block_type=delay
  Delay6 : xbsIndex_r4/Delay  rst=off  infoeditControl=Selection of Reset will increase slice count due to use of real FFs and instead of SRLs  en=off  latency=mult_latency+add_latency+conv_latency  dbl_ovrd=off  reg_retiming=on  block_type=delay
  Delay9 : xbsIndex_r4/Delay  rst=off  infoeditControl=Selection of Reset will increase slice count due to use of real FFs and instead of SRLs  en=off  latency=add_latency+mult_latency+conv_latency  dbl_ovrd=off  reg_retiming=on  block_type=delay
  Reinterpret11 : xbsIndex_r4/Reinterpret  force_arith_type=on  arith_type=Unsigned  force_bin_pt=on  bin_pt=0  block_type=reinterpret
      settings: infoedit="Changes signal type without altering the binary representation.   You can changed the signal between signed and unsigned, and relocate the binary point.<br><br>Hardware notes: In hardware this block costs nothing.<br><br>Example:  Suppose the input is 6 bits wide, signed, with 2 fractional bits, and the output is forced to unsigned with 0 fractional bits.  Then an input of -2.0 (1110.00 in binary 2's complement) becomes an output of 56 (111000 in binary)."  block_version=10.1.3
  c_to_ri : casper_library_misc/c_to_ri  n_bits=data_bit_width  bin_pt=data_bit_width-1
  cmult_dsp48e : casper_library_multipliers/cmult_dsp48e  n_bits_a=18  bin_pt_a=17  n_bits_b=18  bin_pt_b=17  conjugated=off  full_precision=on  n_bits_c=37  bin_pt_c=34  quantization=Truncate  overflow=Wrap  cast_latency=0
      settings: AttributesFormatString=|
      | 18_17 * 18_17 ==> 37_34
      | Latency=4
  polynomial0 : Subsystem  mask(polynomial){order=1, mult_latency=mult_latency, add_latency=add_latency, bit_width_out=lookup_bit_width+fft_len, bin_pt_out=fft_len}
      mask prompts: order "Order of polynomial"; mult_latency "Multiplier latency"; add_latency "Add latency"; bit_width_out "Output bit width"; bin_pt_out "Output binary point"
      settings: AttributesFormatString=latency 6
  ri_to_c : casper_library_misc/ri_to_c
  sincos0 : Subsystem  AncestorBlock=casper_library_downconverter/sincos  mask(sincos){func=sine and cosine, neg_sin=off, neg_cos=off, symmetric=off, handle_sync=on, depth_bits=lookup_bit_width, bit_width=mix_bits, bram_latency=bram_latency}
      mask prompts: func "Function"; neg_sin "Negative sine"; neg_cos "Negative cosine"; symmetric "Symmetric output"; handle_sync "Handle sync"; depth_bits "Lookup table depth (2^?)"; bit_width "Output bit width"; bram_latency "BRAM latency"
      mask init: same as fine_delay_core/fd_fs0/fd_fs0/rotate0/sincos0
      mask TypeOptions func: cosine | sine | sine and cosine
  sync_out : Outport
  dout : Outport  Port=2
  wires:
  polynomial0/2(a0x^0+a1x^1) -> Convert8/1
  polynomial0/1(sync_out) -> Delay13/1
  Reinterpret11/1 -> sincos0/2(theta)
  sincos0/1(sync_out) -> Delay6/1
  cmult_dsp48e/1 -> Convert/1
  cmult_dsp48e/2 -> Convert1/1
  Convert/1 -> ri_to_c/1
  Convert1/1 -> ri_to_c/2
  sincos0/3(cos) -> cmult_dsp48e/1
  sincos0/2(sine) -> cmult_dsp48e/2
  c_to_ri/1 -> Delay10/1
  Delay10/1 -> cmult_dsp48e/3
  c_to_ri/2 -> Delay3/1
  Delay3/1 -> cmult_dsp48e/4
  Delay9/1 -> c_to_ri/1
  Delay13/1 -> sincos0/1(sync_in)
  Convert8/1 -> Reinterpret11/1
  sync/1 -> polynomial0/1(sync_in)
  Delay6/1 -> sync_out/1
  x/1 -> polynomial0/2(x)
  a0/1 -> polynomial0/3(a0)
  a1/1 -> polynomial0/4(a1)
  ri_to_c/1 -> dout/1
  din/1 -> Delay9/1

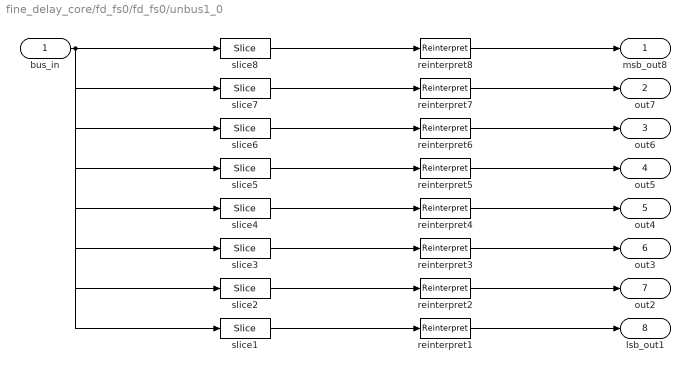
== system fine_delay_core/fd_fs0/fd_fs0/unbus1_0 ==
  bus_in : Inport
  reinterpret{1..8} (8 alike) : xbsIndex_r4/Reinterpret  force_arith_type=on  arith_type=Unsigned  force_bin_pt=on  bin_pt=0  block_type=reinterpret
  slice1 : xbsIndex_r4/Slice  nbits=36  boolean_output=off  mode=Upper Bit Location + Width  bit1=-252  base1=MSB of Input  bit0=0  base0=LSB of Input  dbl_ovrd=off  block_type=slice
  slice2 : xbsIndex_r4/Slice  nbits=36  boolean_output=off  mode=Upper Bit Location + Width  bit1=-216  base1=MSB of Input  bit0=0  base0=LSB of Input  dbl_ovrd=off  block_type=slice
  slice3 : xbsIndex_r4/Slice  nbits=36  boolean_output=off  mode=Upper Bit Location + Width  bit1=-180  base1=MSB of Input  bit0=0  base0=LSB of Input  dbl_ovrd=off  block_type=slice
  slice4 : xbsIndex_r4/Slice  nbits=36  boolean_output=off  mode=Upper Bit Location + Width  bit1=-144  base1=MSB of Input  bit0=0  base0=LSB of Input  dbl_ovrd=off  block_type=slice
  slice5 : xbsIndex_r4/Slice  nbits=36  boolean_output=off  mode=Upper Bit Location + Width  bit1=-108  base1=MSB of Input  bit0=0  base0=LSB of Input  dbl_ovrd=off  block_type=slice
  slice6 : xbsIndex_r4/Slice  nbits=36  boolean_output=off  mode=Upper Bit Location + Width  bit1=-72  base1=MSB of Input  bit0=0  base0=LSB of Input  dbl_ovrd=off  block_type=slice
  slice7 : xbsIndex_r4/Slice  nbits=36  boolean_output=off  mode=Upper Bit Location + Width  bit1=-36  base1=MSB of Input  bit0=0  base0=LSB of Input  dbl_ovrd=off  block_type=slice
  slice8 : xbsIndex_r4/Slice  nbits=36  boolean_output=off  mode=Upper Bit Location + Width  bit1=0  base1=MSB of Input  bit0=0  base0=LSB of Input  dbl_ovrd=off  block_type=slice
  msb_out8 : Outport
  out7 : Outport  Port=2
  out6 : Outport  Port=3
  out5 : Outport  Port=4
  out4 : Outport  Port=5
  out3 : Outport  Port=6
  out2 : Outport  Port=7
  lsb_out1 : Outport  Port=8
  wires:
  bus_in/1 -> slice8/1, slice7/1, slice6/1, slice5/1, slice4/1, slice3/1, slice2/1, slice1/1
  slice8/1 -> reinterpret8/1
  reinterpret8/1 -> msb_out8/1
  slice7/1 -> reinterpret7/1
  reinterpret7/1 -> out7/1
  slice6/1 -> reinterpret6/1
  reinterpret6/1 -> out6/1
  slice5/1 -> reinterpret5/1
  reinterpret5/1 -> out5/1
  slice4/1 -> reinterpret4/1
  reinterpret4/1 -> out4/1
  slice3/1 -> reinterpret3/1
  reinterpret3/1 -> out3/1
  slice2/1 -> reinterpret2/1
  reinterpret2/1 -> out2/1
  slice1/1 -> reinterpret1/1
  reinterpret1/1 -> lsb_out1/1

== system fine_delay_core/fd_fs0/fd_fs0/rotate0/polynomial0 ==
  sync_in : Inport
  x : Inport  Port=2
  a0 : Inport  Port=3
  a1 : Inport  Port=4
  macc : Subsystem  AncestorBlock=casper_library_multipliers/cmult_dsp48e
      settings: AttributesFormatString=|
      | 18_17 * 18_17 ==> 37_34
      | Latency=4
  sync_delay : xbsIndex_r4/Delay  rst=off  infoeditControl=Selection of Reset will increase slice count due to use of real FFs and instead of SRLs  en=off  latency=order*mult_latency+add_latency  dbl_ovrd=off  reg_retiming=on  block_type=delay
  sync_out : Outport
  a0x^0+a1x^1 : Outport  Port=2
  wires:
  a1/1 -> macc/1(a)
  x/1 -> macc/2(b)
  a0/1 -> macc/3(c)
  sync_delay/1 -> sync_out/1
  sync_in/1 -> sync_delay/1
  macc/1(ab_plus_c) -> a0x^0+a1x^1/1

== system fine_delay_core/fd_fs0/fd_fs0/rotate0/sincos0 ==
  sync_in : Inport
  theta : Inport  Port=2
  delay : xbsIndex_r4/Delay  rst=off  infoeditControl=Selection of Reset will increase slice count due to use of real FFs and instead of SRLs  en=off  latency=bram_latency  dbl_ovrd=off  reg_retiming=off  block_type=delay
  rom0 : xbsIndex_r4/ROM  depth=2^depth_bits  initVector=sin(2*pi*(0:(2^depth_bits-1))/(2^depth_bits))  distributed_mem=Block RAM  rst=off  init_reg=0  en=off  latency=bram_latency  gui_display_data_type=Fixed-point  arith_type="Signed  (2's comp)"  n_bits=bit_width  bin_pt=bit_width-1  preci_type=Single  exp_width=8  frac_width=24  dbl_ovrd=off  optimize=Area  use_rpm=on  block_type=sprom
  rom1 : xbsIndex_r4/ROM  depth=2^depth_bits  initVector=cos(2*pi*(0:(2^depth_bits-1))/(2^depth_bits))  distributed_mem=Block RAM  rst=off  init_reg=0  en=off  latency=bram_latency  gui_display_data_type=Fixed-point  arith_type="Signed  (2's comp)"  n_bits=bit_width  bin_pt=bit_width-1  preci_type=Single  exp_width=8  frac_width=24  dbl_ovrd=off  optimize=Area  use_rpm=on  block_type=sprom
  sync_out : Outport
  sine : Outport  Port=2
  cos : Outport  Port=3
  wires:
  sync_in/1 -> delay/1
  delay/1 -> sync_out/1
  theta/1 -> rom0/1, rom1/1
  rom0/1 -> sine/1
  rom1/1 -> cos/1

== system fine_delay_core/fd_fs0/fd_fs0/rotate1/polynomial0 ==
  sync_in : Inport
  x : Inport  Port=2
  a0 : Inport  Port=3
  a1 : Inport  Port=4
  macc : Subsystem  AncestorBlock=casper_library_multipliers/cmult_dsp48e
      settings: AttributesFormatString=|
      | 18_17 * 18_17 ==> 37_34
      | Latency=4
  sync_delay : xbsIndex_r4/Delay  rst=off  infoeditControl=Selection of Reset will increase slice count due to use of real FFs and instead of SRLs  en=off  latency=order*mult_latency+add_latency  dbl_ovrd=off  reg_retiming=on  block_type=delay
  sync_out : Outport
  a0x^0+a1x^1 : Outport  Port=2
  wires:
  macc/1(ab_plus_c) -> a0x^0+a1x^1/1
  sync_in/1 -> sync_delay/1
  sync_delay/1 -> sync_out/1
  a0/1 -> macc/3(c)
  x/1 -> macc/2(b)
  a1/1 -> macc/1(a)

== system fine_delay_core/fd_fs0/fd_fs0/rotate1/sincos0 ==
  sync_in : Inport
  theta : Inport  Port=2
  delay : xbsIndex_r4/Delay  rst=off  infoeditControl=Selection of Reset will increase slice count due to use of real FFs and instead of SRLs  en=off  latency=bram_latency  dbl_ovrd=off  reg_retiming=off  block_type=delay
  rom0 : xbsIndex_r4/ROM  depth=2^depth_bits  initVector=sin(2*pi*(0:(2^depth_bits-1))/(2^depth_bits))  distributed_mem=Block RAM  rst=off  init_reg=0  en=off  latency=bram_latency  gui_display_data_type=Fixed-point  arith_type="Signed  (2's comp)"  n_bits=bit_width  bin_pt=bit_width-1  preci_type=Single  exp_width=8  frac_width=24  dbl_ovrd=off  optimize=Area  use_rpm=on  block_type=sprom
  rom1 : xbsIndex_r4/ROM  depth=2^depth_bits  initVector=cos(2*pi*(0:(2^depth_bits-1))/(2^depth_bits))  distributed_mem=Block RAM  rst=off  init_reg=0  en=off  latency=bram_latency  gui_display_data_type=Fixed-point  arith_type="Signed  (2's comp)"  n_bits=bit_width  bin_pt=bit_width-1  preci_type=Single  exp_width=8  frac_width=24  dbl_ovrd=off  optimize=Area  use_rpm=on  block_type=sprom
  sync_out : Outport
  sine : Outport  Port=2
  cos : Outport  Port=3
  wires:
  rom1/1 -> cos/1
  rom0/1 -> sine/1
  theta/1 -> rom1/1, rom0/1
  delay/1 -> sync_out/1
  sync_in/1 -> delay/1
